simulink model "yumiao_SMC_motor_10"  (Simulink 8.4)
settings: Solver=ode45  StartTime=0.0  StopTime=223.5  RelTol=1e-3
libraries: simulink x3, Solver_SF x1
settings Model: Creator=强哥  LastModifiedBy=强哥
settings DataIOCC: SignalLoggingSaveFormat=Dataset
settings OptimizationCC: ExpressionDepthLimit=128
settings DebuggingCC: UnderspecifiedInitializationDetection=Simplified  MergeDetectMultiDrivingBlocksExec=error  FcnCallInpInsideContextMsg=EnableAllAsError  StateNameClashWarn=none
settings GRTTargetCC: CombineOutputUpdateFcns=on  GRTInterface=off

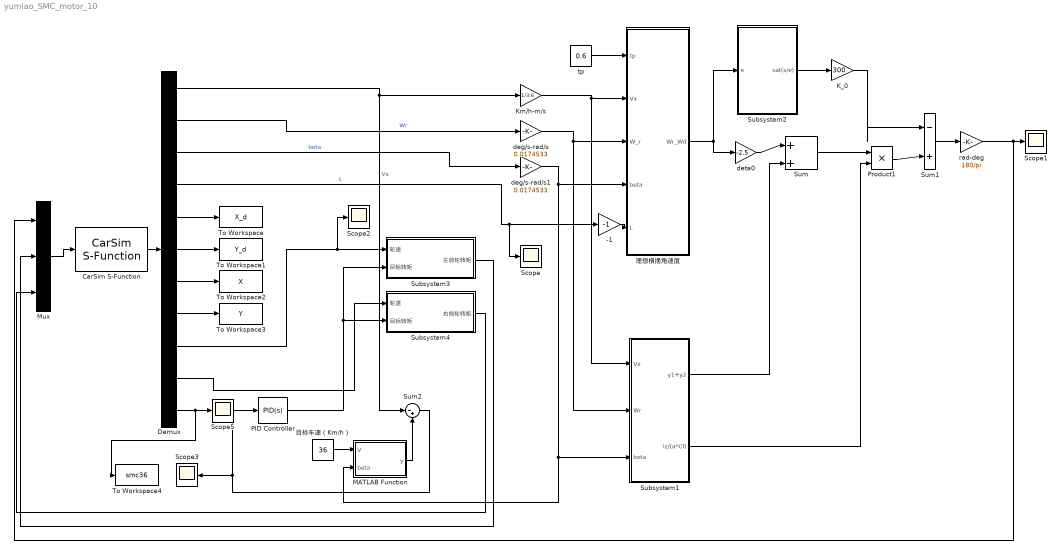
== system yumiao_SMC_motor_10 ==
  "-1 " : Gain  Gain=-1
  CarSim S-Function : Solver_SF/CarSim S-Function  Priority=1  VehicleCode=i_i  SIMFILE=simfile
  Demux : Demux  Outputs=11
  K_0 : Gain  Gain=300
  Km/h-m/s : Gain  Gain=1/3.6
  MATLAB Function : MATLAB Function  TreatAsAtomicUnit=on
  Mux : Mux  Inputs=3
  PID Controller : simulink/Continuous/PID Controller  Controller=PID  TimeDomain=Continuous-time  SampleTime=-1  IntegratorMethod=Forward Euler  FilterMethod=Forward Euler  Form=Parallel  P=200  I=190  D=2  N=100  InitialConditionSource=internal  InitialConditionForIntegrator=0  InitialConditionForFilter=0  ExternalReset=none  LimitOutput=off  UpperSaturationLimit=inf  LowerSaturationLimit=-inf  LinearizeAsGain=on  AntiWindupMode=none  Kb=1  TrackingMode=off  Kt=1  PParamMin=[]  PParamMax=[]  IParamMin=[]  IParamMax=[]  DParamMin=[]  DParamMax=[]  NParamMin=[]  NParamMax=[]  KbParamMin=[]  KbParamMax=[]  KtParamMin=[]  KtParamMax=[]  POutMin=[]  POutMax=[]  IOutMin=[]  IOutMax=[]  DOutMin=[]  DOutMax=[]  NOutMin=[]  NOutMax=[]  KbOutMin=[]  KbOutMax=[]  KtOutMin=[]  KtOutMax=[]  IntegratorOutMin=[]  IntegratorOutMax=[]  FilterOutMin=[]  FilterOutMax=[]  SumOutMin=[]  SumOutMax=[]  SumI1OutMin=[]  SumI1OutMax=[]  SumI2OutMin=[]  SumI2OutMax=[]  SumI3OutMin=[]  SumI3OutMax=[]  SumDOutMin=[]  SumDOutMax=[]  SaturationOutMin=[]  SaturationOutMax=[]  IntegratorContinuousStateAttributes=''  IntegratorStateMustResolveToSignalObject=off  IntegratorRTWStateStorageClass=Auto  FilterContinuousStateAttributes=''  FilterStateMustResolveToSignalObject=off  FilterRTWStateStorageClass=Auto  DifferentiatorICPrevScaledInput=0  DifferentiatorOutMin=[]  DifferentiatorOutMax=[]  UseFilter=on
  Product1 : Product
  Scope{,1..3,5} (5 alike) : Scope
      Scope settings: TimeRange=80  YMin=-0.15  YMax=0.15
      Scope2 settings: TimeRange=80  YMin=-0.15  YMax=0.15  SaveName=ScopeData2
      Scope3 settings: TimeRange=80  YMin=-0.15  YMax=0.15  SaveName=ScopeData3
      Scope5 settings: TimeRange=80  YMin=-0.2  YMax=0.2  SaveName=ScopeData5
  Subsystem1 : Subsystem
  Subsystem2 : Subsystem
  Subsystem3 : Subsystem
  Subsystem4 : Subsystem
  Sum : Sum  Inputs=|++
  Sum1 : Sum  Inputs=|-+
  Sum2 : Sum  Inputs=|-+
  To Workspace : ToWorkspace  VariableName=X_d  SampleTime=-1
  To Workspace1 : ToWorkspace  VariableName=Y_d  SampleTime=-1
  To Workspace2 : ToWorkspace  VariableName=X  SampleTime=-1
  To Workspace3 : ToWorkspace  VariableName=Y  SampleTime=-1
  To Workspace4 : ToWorkspace  VariableName=smc36  SampleTime=-1
  deg/s-rad/s : Gain  Gain=0.0174533
  deg/s-rad/s1 : Gain  Gain=0.0174533
  deta0 : Gain  Gain=-2.5
  rad-deg : Gain  Gain=180/pi
  tp : Constant  Value=0.6
  理想横摆角速度 : Subsystem
  目标车速（Km/h） : Constant  Value=36
  wires:
  Demux/1 -> Km/h-m/s/1, Sum2/1  "Vx"
  Demux/2 -> deg/s-rad/s/1  "Wr"
  Demux/3 -> deg/s-rad/s1/1  "beta"
  Demux/4 -> "-1 "/1, Scope/1  "L"
  Km/h-m/s/1 -> 理想横摆角速度/2(Vx), Subsystem1/1(Vx)
  tp/1 -> 理想横摆角速度/1(tp)
  deg/s-rad/s/1 -> 理想横摆角速度/3(W_r), Subsystem1/2(Wr)
  deg/s-rad/s1/1 -> 理想横摆角速度/4(beta), Subsystem1/3(beta), MATLAB Function/2(beta)
  理想横摆角速度/1(Wr_Wd) -> Subsystem2/1(e), deta0/1
  deta0/1 -> Sum/1
  Subsystem1/1(y1+y2) -> Sum/2
  Sum/1 -> Product1/1
  Subsystem1/2(Iz/(a*Cf)) -> Product1/2
  Subsystem2/1(sat(s/e)) -> K_0/1
  Product1/1 -> Sum1/2
  K_0/1 -> Sum1/1
  Sum1/1 -> rad-deg/1
  rad-deg/1 -> Scope1/1, Mux/1
  "-1 "/1 -> 理想横摆角速度/5(L)
  Demux/5 -> To Workspace/1
  Demux/6 -> To Workspace1/1
  Demux/7 -> To Workspace2/1
  Demux/8 -> To Workspace3/1
  Demux/9 -> Scope2/1, Subsystem3/1(轮速)
  Demux/10 -> Subsystem4/1(轮速)
  PID Controller/1 -> Subsystem3/2(目标转矩), Subsystem4/2(目标转矩)
  目标车速（Km/h）/1 -> MATLAB Function/1(V)
  MATLAB Function/1(y) -> Sum2/2
  Sum2/1 -> Scope3/1, PID Controller/1
  Subsystem3/1("左前轮转矩 ") -> Mux/2
  Subsystem4/1("右前轮转矩 ") -> Mux/3
  Mux/1 -> CarSim S-Function/1
  CarSim S-Function/1 -> Demux/1
  Demux/11 -> To Workspace4/1, Scope5/1

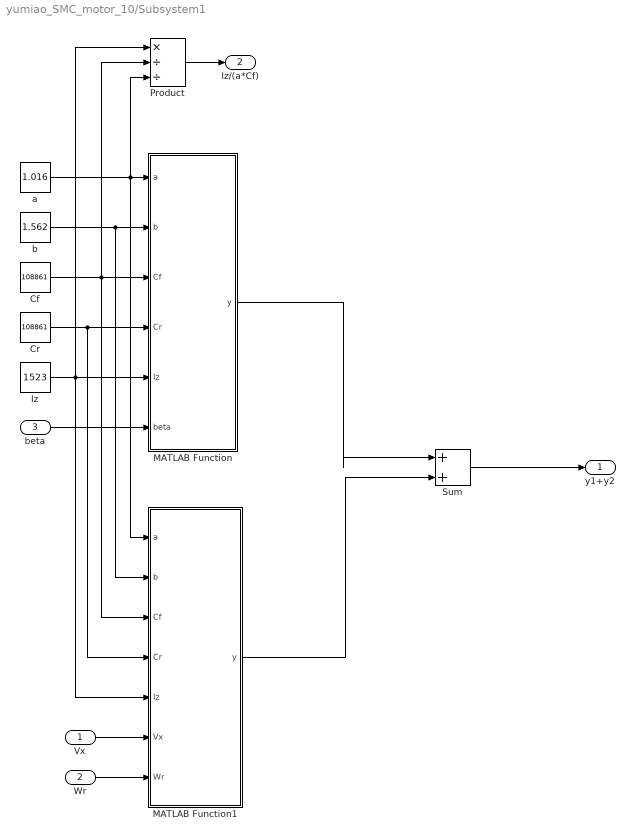
== system yumiao_SMC_motor_10/Subsystem1 ==
  Vx : Inport
  Wr : Inport  Port=2
  beta : Inport  Port=3
  Cf : Constant  Value=108861
  Cr : Constant  Value=108861
  Iz : Constant  Value=1523
  MATLAB Function : MATLAB Function  TreatAsAtomicUnit=on
  MATLAB Function1 : MATLAB Function  TreatAsAtomicUnit=on
  Product : Product  Inputs=*//
  Sum : Sum  Inputs=|++
  a : Constant  Value=1.016
  b : Constant  Value=1.562
  y1+y2 : Outport
  Iz/(a*Cf) : Outport  Port=2
  wires:
  a/1 -> MATLAB Function1/1(a), Product/3, MATLAB Function/1(a)
  b/1 -> MATLAB Function1/2(b), MATLAB Function/2(b)
  Cf/1 -> Product/2, MATLAB Function1/3(Cf), MATLAB Function/3(Cf)
  Cr/1 -> MATLAB Function1/4(Cr), MATLAB Function/4(Cr)
  Iz/1 -> Product/1, MATLAB Function1/5(Iz), MATLAB Function/5(Iz)
  beta/1 -> MATLAB Function/6(beta)
  Vx/1 -> MATLAB Function1/6(Vx)
  Wr/1 -> MATLAB Function1/7(Wr)
  MATLAB Function/1(y) -> Sum/1
  MATLAB Function1/1(y) -> Sum/2
  Sum/1 -> y1+y2/1
  Product/1 -> Iz/(a*Cf)/1

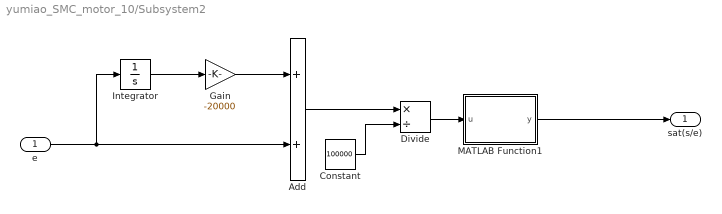
== system yumiao_SMC_motor_10/Subsystem2 ==
  e : Inport
  Add : Sum
  Constant : Constant  Value=100000
  Divide : Product  Inputs=*/
  Gain : Gain  Gain=-20000
  Integrator : Integrator
  MATLAB Function1 : MATLAB Function  TreatAsAtomicUnit=on
  sat(s/e) : Outport
  wires:
  Integrator/1 -> Gain/1
  MATLAB Function1/1(y) -> sat(s/e)/1
  Gain/1 -> Add/1
  Add/1 -> Divide/1
  e/1 -> Integrator/1, Add/2
  Constant/1 -> Divide/2
  Divide/1 -> MATLAB Function1/1(u)

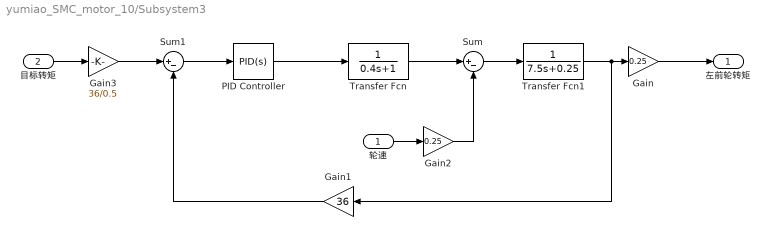
== system yumiao_SMC_motor_10/Subsystem3 ==
  轮速 : Inport
  目标转矩 : Inport  Port=2
  Gain : Gain  Gain=0.25
  Gain1 : Gain  Gain=36
  Gain2 : Gain  Gain=0.25
  Gain3 : Gain  Gain=36/0.5
  PID Controller : simulink/Continuous/PID Controller  Controller=PID  TimeDomain=Continuous-time  SampleTime=-1  IntegratorMethod=Forward Euler  FilterMethod=Forward Euler  Form=Parallel  P=200  I=30  D=2  N=100  InitialConditionSource=internal  InitialConditionForIntegrator=0  InitialConditionForFilter=0  ExternalReset=none  LimitOutput=off  UpperSaturationLimit=inf  LowerSaturationLimit=-inf  LinearizeAsGain=on  AntiWindupMode=none  Kb=1  TrackingMode=off  Kt=1  PParamMin=[]  PParamMax=[]  IParamMin=[]  IParamMax=[]  DParamMin=[]  DParamMax=[]  NParamMin=[]  NParamMax=[]  KbParamMin=[]  KbParamMax=[]  KtParamMin=[]  KtParamMax=[]  POutMin=[]  POutMax=[]  IOutMin=[]  IOutMax=[]  DOutMin=[]  DOutMax=[]  NOutMin=[]  NOutMax=[]  KbOutMin=[]  KbOutMax=[]  KtOutMin=[]  KtOutMax=[]  IntegratorOutMin=[]  IntegratorOutMax=[]  FilterOutMin=[]  FilterOutMax=[]  SumOutMin=[]  SumOutMax=[]  SumI1OutMin=[]  SumI1OutMax=[]  SumI2OutMin=[]  SumI2OutMax=[]  SumI3OutMin=[]  SumI3OutMax=[]  SumDOutMin=[]  SumDOutMax=[]  SaturationOutMin=[]  SaturationOutMax=[]  IntegratorContinuousStateAttributes=''  IntegratorStateMustResolveToSignalObject=off  IntegratorRTWStateStorageClass=Auto  FilterContinuousStateAttributes=''  FilterStateMustResolveToSignalObject=off  FilterRTWStateStorageClass=Auto  DifferentiatorICPrevScaledInput=0  DifferentiatorOutMin=[]  DifferentiatorOutMax=[]  UseFilter=on
  Sum : Sum  Inputs=|+-
  Sum1 : Sum  Inputs=|+-
  Transfer Fcn : TransferFcn  Denominator=[0.4 1]
  Transfer Fcn1 : TransferFcn  Denominator=[7.5 0.25]
  "左前轮转矩 " : Outport
  wires:
  PID Controller/1 -> Transfer Fcn/1
  Transfer Fcn/1 -> Sum/1
  Sum/1 -> Transfer Fcn1/1
  Transfer Fcn1/1 -> Gain1/1, Gain/1
  Gain/1 -> "左前轮转矩 "/1
  目标转矩/1 -> Gain3/1
  Sum1/1 -> PID Controller/1
  Gain1/1 -> Sum1/2
  轮速/1 -> Gain2/1
  Gain2/1 -> Sum/2
  Gain3/1 -> Sum1/1

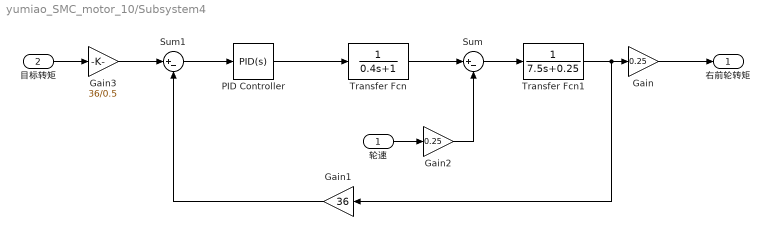
== system yumiao_SMC_motor_10/Subsystem4 ==
  轮速 : Inport
  目标转矩 : Inport  Port=2
  Gain : Gain  Gain=0.25
  Gain1 : Gain  Gain=36
  Gain2 : Gain  Gain=0.25
  Gain3 : Gain  Gain=36/0.5
  PID Controller : simulink/Continuous/PID Controller  Controller=PID  TimeDomain=Continuous-time  SampleTime=-1  IntegratorMethod=Forward Euler  FilterMethod=Forward Euler  Form=Parallel  P=200  I=30  D=2  N=100  InitialConditionSource=internal  InitialConditionForIntegrator=0  InitialConditionForFilter=0  ExternalReset=none  LimitOutput=off  UpperSaturationLimit=inf  LowerSaturationLimit=-inf  LinearizeAsGain=on  AntiWindupMode=none  Kb=1  TrackingMode=off  Kt=1  PParamMin=[]  PParamMax=[]  IParamMin=[]  IParamMax=[]  DParamMin=[]  DParamMax=[]  NParamMin=[]  NParamMax=[]  KbParamMin=[]  KbParamMax=[]  KtParamMin=[]  KtParamMax=[]  POutMin=[]  POutMax=[]  IOutMin=[]  IOutMax=[]  DOutMin=[]  DOutMax=[]  NOutMin=[]  NOutMax=[]  KbOutMin=[]  KbOutMax=[]  KtOutMin=[]  KtOutMax=[]  IntegratorOutMin=[]  IntegratorOutMax=[]  FilterOutMin=[]  FilterOutMax=[]  SumOutMin=[]  SumOutMax=[]  SumI1OutMin=[]  SumI1OutMax=[]  SumI2OutMin=[]  SumI2OutMax=[]  SumI3OutMin=[]  SumI3OutMax=[]  SumDOutMin=[]  SumDOutMax=[]  SaturationOutMin=[]  SaturationOutMax=[]  IntegratorContinuousStateAttributes=''  IntegratorStateMustResolveToSignalObject=off  IntegratorRTWStateStorageClass=Auto  FilterContinuousStateAttributes=''  FilterStateMustResolveToSignalObject=off  FilterRTWStateStorageClass=Auto  DifferentiatorICPrevScaledInput=0  DifferentiatorOutMin=[]  DifferentiatorOutMax=[]  UseFilter=on
  Sum : Sum  Inputs=|+-
  Sum1 : Sum  Inputs=|+-
  Transfer Fcn : TransferFcn  Denominator=[0.4 1]
  Transfer Fcn1 : TransferFcn  Denominator=[7.5 0.25]
  "右前轮转矩 " : Outport
  wires:
  PID Controller/1 -> Transfer Fcn/1
  Transfer Fcn/1 -> Sum/1
  Sum/1 -> Transfer Fcn1/1
  Transfer Fcn1/1 -> Gain1/1, Gain/1
  Gain/1 -> "右前轮转矩 "/1
  目标转矩/1 -> Gain3/1
  Sum1/1 -> PID Controller/1
  Gain1/1 -> Sum1/2
  轮速/1 -> Gain2/1
  Gain2/1 -> Sum/2
  Gain3/1 -> Sum1/1

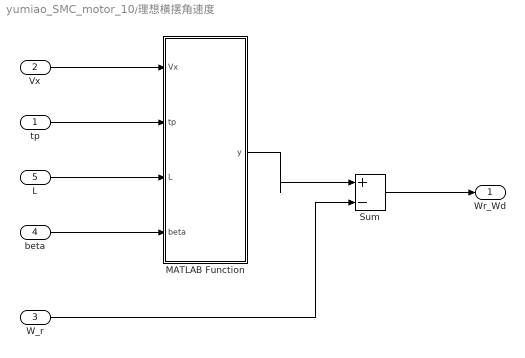
== system yumiao_SMC_motor_10/理想横摆角速度 ==
  tp : Inport
  Vx : Inport  Port=2
  W_r : Inport  Port=3
  beta : Inport  Port=4
  L : Inport  Port=5
  MATLAB Function : MATLAB Function  TreatAsAtomicUnit=on
  Sum : Sum  Inputs=|+-
  Wr_Wd : Outport
  wires:
  Vx/1 -> MATLAB Function/1(Vx)
  tp/1 -> MATLAB Function/2(tp)
  L/1 -> MATLAB Function/3(L)
  beta/1 -> MATLAB Function/4(beta)
  MATLAB Function/1(y) -> Sum/1
  W_r/1 -> Sum/2
  Sum/1 -> Wr_Wd/1

== matlab function Subsystem1/MATLAB Function ==
  data: a input double; y output double; b input double; Cf input double; Cr input double; Iz input double; beta input double
function y = fcn(a,b,Cf,Cr,Iz,beta)
%#codegen

y = beta*(a*Cf-b*Cr)/Iz;

== matlab function 理想横摆角速度/MATLAB Function ==
  data: Vx input double; y output double; tp input double; L input double; beta input double
function y = fcn(Vx,tp,L,beta)
%#codegen

y = 2*(atan(L/(Vx*tp))-beta)/tp;

== matlab function Subsystem1/MATLAB Function1 ==
  data: a input double; y output double; b input double; Cf input double; Cr input double; Iz input double; Vx input double; Wr input double
function y = fcn(a,b,Cf,Cr,Iz,Vx,Wr)
%#codegen

y =Wr*(Cf*a^2+Cr*b^2)/(Iz*Vx);

== matlab function Subsystem2/MATLAB Function1 ==
  data: u input double; y output double
function y = fcn(u)
if abs(u)<=1;
    y=u;
else
y =sign(u);
end

== matlab function MATLAB Function ==
  data: V input double; beta input double; y output double
function y = fcn(V,beta)
%#codegen

y = V*cos(beta);
